simulink model "Motor610"  (Simulink 8.3)
settings: Solver=ode45  SolverMode=SingleTasking  StartTime=0.0  StopTime=20  RelTol=1e-3
values from neighbouring files (symbols this model uses):
  power_max = 80000    [Motor.m]
  Tc = 0.02    [Motor.m]
  torque_max = 280    [Motor.m]
  x_losses_mat = [3.1 2.21 1.67 1.49 1.67 2.31 3.1;2.03 1.14 0.69 0.42 0.69 1.14 2.03;1.68 0.78 0.24 0.06 0.24 0.78 1.68;2.03 1.14 0.69 0.42 0.69 1.14 2.03;3.1 2.21 1.67 1.49 1.67 2.21 3.1]    [Motor.m]
  x_T_eff_vec = [-0.09 -0.06 -0.03 0 0.03 0.06 0.09]    [Motor.m]
  x_w_eff_vec = [-8000 -4000 0 4000 8000]    [Motor.m]
settings Model: Creator=xiaom  LastModifiedBy=xiaom  CovMetricSettings=dwe  CovHtmlReporting=off  covSaveCumulativeToWorkspaceVar=off  CovSaveSingleToWorkspaceVar=off  CovExternalEMLEnable=on  CovSFcnEnable=on
settings DataIOCC: LimitDataPoints=off  SaveFormat=StructureWithTime  SignalLoggingSaveFormat=Dataset
settings DebuggingCC: UnderspecifiedInitializationDetection=Simplified  MergeDetectMultiDrivingBlocksExec=error  SolverPrmCheckMsg=none  FrameProcessingCompatibilityMsg=error  StateNameClashWarn=none  SFUnexpectedBacktrackingDiag=error  SFNoUnconditionalDefaultTransitionDiag=error
settings HardwareCC: ProdBitPerPointer=64  ProdLargestAtomicFloat=Float  ProdIntDivRoundTo=Zero  ProdEndianess=LittleEndian  ProdHWDeviceType=Specified
settings ModelReferenceCC: PropagateSignalLabelsOutOfModel=on
settings SFSimCC: SimUseLocalCustomCode=on
settings RTWCC: RTWUseLocalCustomCode=on
settings GRTTargetCC: TargetLangStandard=C99 (ISO)  GeneratePreprocessorConditionals=Use local settings  CombineOutputUpdateFcns=on  GRTInterface=off

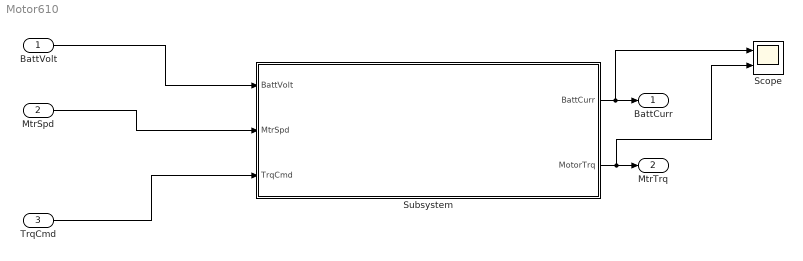
== system Motor610 ==
  BattVolt : Inport
  MtrSpd : Inport  Port=2
  TrqCmd : Inport  Port=3
  Scope : Scope  NumInputPorts=2
      settings: TimeRange=auto  MaxDataPoints=5000  SaveToWorkspace=off  SaveName=ScopeData  YMin=-36.83014~-36.83014  YMax=331.47128~331.47128  SampleTime=-1
  Subsystem : Subsystem
  BattCurr : Outport
  MtrTrq : Outport  Port=2
  wires:
  Subsystem/2(MotorTrq) -> Scope/2, MtrTrq/1
  Subsystem/1(BattCurr) -> Scope/1, BattCurr/1
  MtrSpd/1 -> Subsystem/2(MtrSpd)
  BattVolt/1 -> Subsystem/1(BattVolt)
  TrqCmd/1 -> Subsystem/3(TrqCmd)

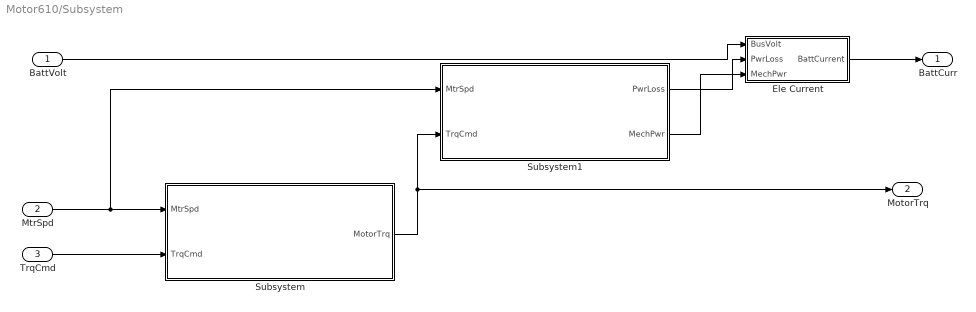
== system Motor610/Subsystem ==
  BattVolt : Inport
  MtrSpd : Inport  Port=2
  TrqCmd : Inport  Port=3
  Ele Current : Subsystem
  Subsystem : Subsystem
  Subsystem1 : Subsystem
  BattCurr : Outport
  MotorTrq : Outport  Port=2
  wires:
  MtrSpd/1 -> Subsystem1/1(MtrSpd), Subsystem/1(MtrSpd)
  BattVolt/1 -> Ele Current/1(BusVolt)
  TrqCmd/1 -> Subsystem/2(TrqCmd)
  Subsystem/1(MotorTrq) -> MotorTrq/1, Subsystem1/2(TrqCmd)
  Subsystem1/1(PwrLoss) -> Ele Current/2(PwrLoss)
  Subsystem1/2(MechPwr) -> Ele Current/3(MechPwr)
  Ele Current/1(BattCurrent) -> BattCurr/1

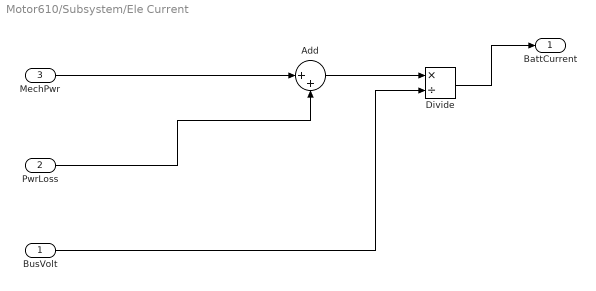
== system Motor610/Subsystem/Ele Current ==
  BusVolt : Inport
  PwrLoss : Inport  Port=2
  MechPwr : Inport  Port=3
  Add : Sum  Inputs=|++
  Divide : Product  Inputs=*/
  BattCurrent : Outport
  wires:
  PwrLoss/1 -> Add/2
  BusVolt/1 -> Divide/2
  MechPwr/1 -> Add/1
  Add/1 -> Divide/1
  Divide/1 -> BattCurrent/1

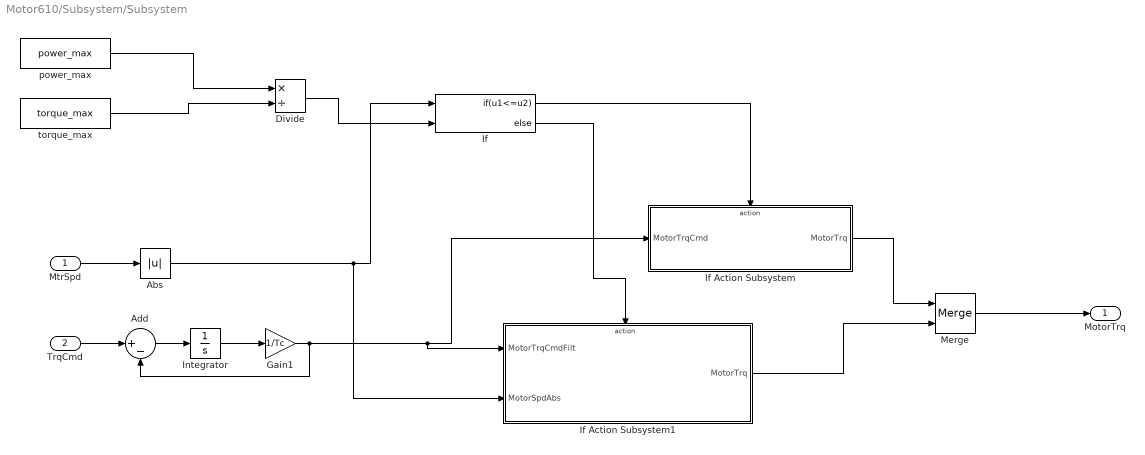
== system Motor610/Subsystem/Subsystem ==
  MtrSpd : Inport
  TrqCmd : Inport  Port=2
  Abs : Abs
  Add : Sum  Inputs=|+-
  Divide : Product  Inputs=*/  SaturateOnIntegerOverflow=on  RndMeth=Zero
  Gain1 : Gain  Gain=1/Tc
  If : If  NumInputs=2  IfExpression=u1<=u2
  If Action Subsystem : Subsystem  TreatAsAtomicUnit=on
  If Action Subsystem1 : Subsystem  TreatAsAtomicUnit=on
  Integrator : Integrator
  Merge : Merge
  power_max : Constant  Value=power_max
  torque_max : Constant  Value=torque_max
  MotorTrq : Outport
  wires:
  MtrSpd/1 -> Abs/1
  Add/1 -> Integrator/1
  power_max/1 -> Divide/1
  torque_max/1 -> Divide/2
  Divide/1 -> If/2
  Abs/1 -> If Action Subsystem1/2(MotorSpdAbs), If/1
  If/1 -> If Action Subsystem/Action
  If/2 -> If Action Subsystem1/Action
  TrqCmd/1 -> Add/1
  Integrator/1 -> Gain1/1
  Gain1/1 -> If Action Subsystem1/1(MotorTrqCmdFilt), If Action Subsystem/1(MotorTrqCmd), Add/2
  If Action Subsystem/1(MotorTrq) -> Merge/1
  If Action Subsystem1/1(MotorTrq) -> Merge/2
  Merge/1 -> MotorTrq/1

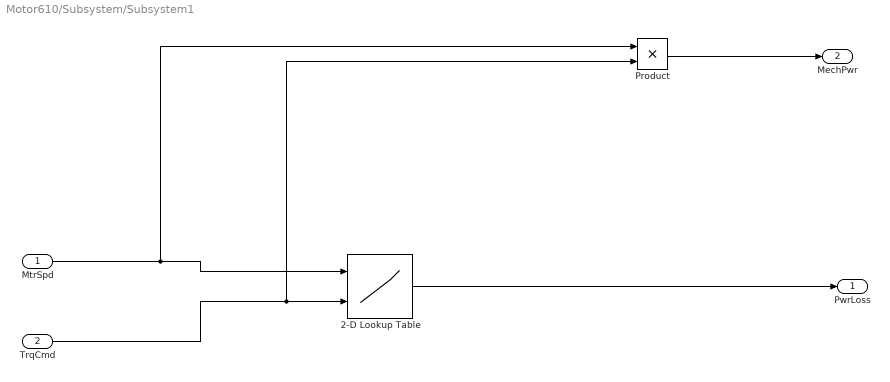
== system Motor610/Subsystem/Subsystem1 ==
  MtrSpd : Inport
  TrqCmd : Inport  Port=2
  2-D Lookup Table : Lookup_n-D  BreakpointsForDimension1=x_w_eff_vec  BreakpointsForDimension2=x_T_eff_vec  Table=x_losses_mat  InternalRulePriority=Speed  RndMeth=Simplest  InputSameDT=on
  Product : Product
  PwrLoss : Outport
  MechPwr : Outport  Port=2
  wires:
  MtrSpd/1 -> Product/1, 2-D Lookup Table/1
  TrqCmd/1 -> Product/2, 2-D Lookup Table/2
  2-D Lookup Table/1 -> PwrLoss/1
  Product/1 -> MechPwr/1

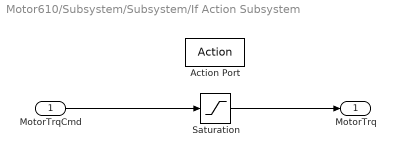
== system Motor610/Subsystem/Subsystem/If Action Subsystem ==
  MotorTrqCmd : Inport
  Action Port : ActionPort  ActionType=then
  Saturation : Saturate  UpperLimit=torque_max  LowerLimit=-torque_max
  MotorTrq : Outport
  wires:
  MotorTrqCmd/1 -> Saturation/1
  Saturation/1 -> MotorTrq/1

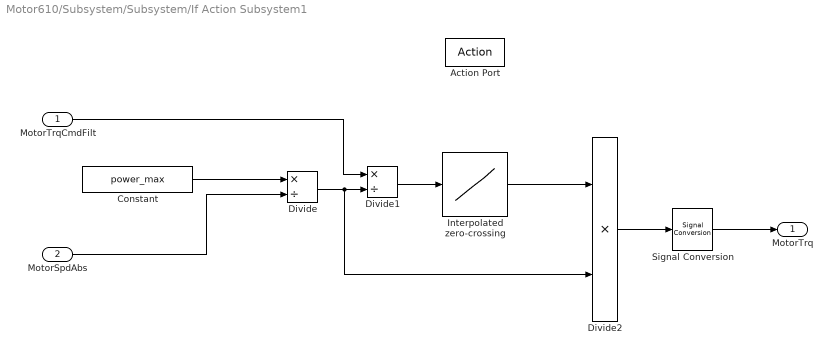
== system Motor610/Subsystem/Subsystem/If Action Subsystem1 ==
  MotorTrqCmdFilt : Inport
  MotorSpdAbs : Inport  Port=2
  Action Port : ActionPort  ActionType=else
  Constant : Constant  Value=power_max
  Divide : Product  Inputs=*/
  Divide1 : Product  Inputs=*/
  Divide2 : Product
  Interpolated zero-crossing : Lookup_n-D  NumberOfTableDimensions=1  BreakpointsForDimension1=[-1 1]  Table=[-1 1]  ExtrapMethod=Clip  InternalRulePriority=Speed  RndMeth=Simplest  InputSameDT=on
  Signal Conversion : SignalConversion  OverrideOpt=off
  MotorTrq : Outport  InitialOutput=0
  wires:
  MotorTrqCmdFilt/1 -> Divide1/1
  Divide/1 -> Divide1/2, Divide2/2
  Divide1/1 -> Interpolated zero-crossing/1
  Interpolated zero-crossing/1 -> Divide2/1
  Divide2/1 -> Signal Conversion/1
  Constant/1 -> Divide/1
  Signal Conversion/1 -> MotorTrq/1
  MotorSpdAbs/1 -> Divide/2
